simulink model "AE_BoltEV_LMDI"  (R2026a)
settings: Solver=ode23t  StartTime=0  StopTime=1800  FixedStep=Ts  MaxStep=0.01  EnableMultiTasking=on
InitFcn:
  | AE_BoltEV_LMDI_Params;
undefined symbols (not defined in the file): id_map, iq_map, Is_map, n_loss_bp, P, P_cu_map, P_iron_map, T_loss_bp, Tmax, V_oc
libraries: nesl_utility x14, fl_lib x12, autolibshared x2, sdl_lib x2, autolibmappedmotor x1, sl_discontinuities x1
(part 2 of 3)

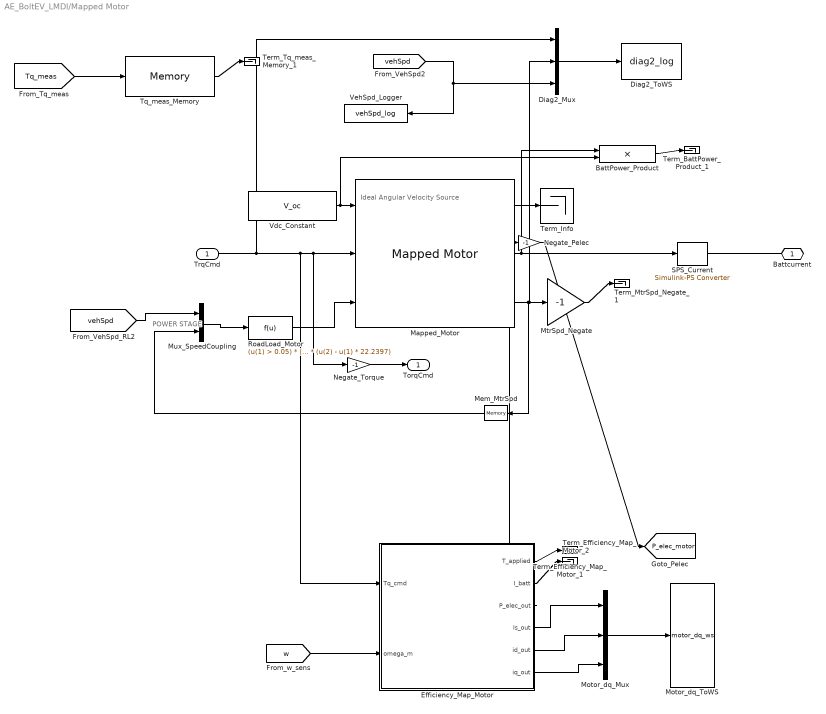
== system AE_BoltEV_LMDI/Mapped Motor ==
  note: Ideal Angular Velocity Source
  note: POWER STAGE
  TrqCmd : Inport
  BattPower_Product : Product
  Diag2_Mux : Mux  Inputs=3
  Diag2_ToWS : ToWorkspace  VariableName=diag2_log  SampleTime=0.1
  Efficiency_Map_Motor : Subsystem  Description=Efficiency-map motor. P_elec = sign(Tw)(|Tw| + P_loss). Bolt EV 150 kW IPM.
  Mapped_Motor : autolibmappedmotor/Mapped Motor  w_Tmax_bp_ext=[-921.533845053006 -837.758040957278 -785.398163397448 -733.038285837618 -680.678408277789 -628.318530717959 -575.958653158129 -523.598775598299 -460.766922526503 -366.519142918809 -0.10471975511966 0 0.10471975511966 366.519142918809 460.766922526503 523.598775598299 575.958653158129 628.318530717959 680.678408277789 733.038285837618 785.398163397448 837.758040957278 921.533845053006]  Tmax_w_V_ext=[162 162 162;179 179 179;191 191 191;204 204 204;220 220 220;238 238 238;260 260 260;286 286 286;325 325 325;360 360 360;360 360 360;360 360 360;360 360 360;360 360 360;325 325 325;286 286 286;260 260 260;238 238 238;220 220 220;204 204 204;191 191 191;179 179 179;162 162 162]  w_Tmin_bp_ext=[-921.533845053006 -837.758040957278 -785.398163397448 -733.038285837618 -680.678408277789 -628.318530717959 -575.958653158129 -523.598775598299 -460.766922526503 -366.519142918809 -0.10471975511966 0 0.10471975511966 366.519142918809 460.766922526503 523.598775598299 575.958653158129 628.318530717959 680.678408277789 733.038285837618 785.398163397448 837.758040957278 921.533845053006]  Tmin_w_V_ext=[-162 -162 -162;-179 -179 -179;-191 -191 -191;-204 -204 -204;-220 -220 -220;-238 -238 -238;-260 -260 -260;-286 -286 -286;-325 -325 -325;-360 -360 -360;-360 -360 -360;-360 -360 -360;-360 -360 -360;-360 -360 -360;-325 -325 -325;-286 -286 -286;-260 -260 -260;-238 -238 -238;-220 -220 -220;-204 -204 -204;-191 -191 -191;-179 -179 -179;-162 -162 -162]  port_config=Torque  param_by=Tabulated torque-speed envelope  w_t=[0 0.10471975511966 366.519142918809 460.766922526503 523.598775598299 575.958653158129 628.318530717959 680.678408277789 733.038285837618 785.398163397448 837.758040957278 921.533845053006]  T_t=[360 360 360 325 286 260 238 220 204 191 179 162]  torque_max=360  power_max=150  SpreadsheetTqLimitsFileName=MotorCalibrationImportData.xlsx  Tmax_w_V=[360 360 360;360 360 360;360 360 360;325 325 325;286 286 286;260 260 260;238 238 238;220 220 220;204 204 204;191 191 191;179 179 179;162 162 162]  w_Tmax_bp=[0 0.10471975511966 366.519142918809 460.766922526503 523.598775598299 575.958653158129 628.318530717959 680.678408277789 733.038285837618 785.398163397448 837.758040957278 921.533845053006]  V_Tmax_bp=[300 380 420]  Tmin_w_V=[-360 -360 -360;-360 -360 -360;-360 -360 -360;-325 -325 -325;-286 -286 -286;-260 -260 -260;-238 -238 -238;-220 -220 -220;-204 -204 -204;-191 -191 -191;-179 -179 -179;-162 -162 -162]  w_Tmin_bp=[0 0.10471975511966 366.519142918809 460.766922526503 523.598775598299 575.958653158129 628.318530717959 680.678408277789 733.038285837618 785.398163397448 837.758040957278 921.533845053006]  V_Tmin_bp=[300 380 420]  Tc=0.02  param_loss=Tabulated loss data  SpreadsheetLossFileName=MotorCalibrationImportData.xlsx  SpreadsheetEffFileName=MotorCalibrationImportData.xlsx  eff=100  w_eff=375  T_eff=0.08  Piron=0  Pbase=0  w_eff_bp=[10.472 31.4159 52.3599 73.3038 94.2478 115.192 136.136 157.08 178.024 198.968 219.911 240.855 261.799 282.743 303.687 324.631 345.575 366.519 387.463 408.407 429.351 450.295 471.239 492.183 513.127 534.071 555.015 575.959 596.903 617.847 638.791 659.734 680.678 701.622 722.566 743.51 764.454 785.398 806.342 827.286 848.23 869.174 890.118 911.062]  T_eff_bp=[5 15 25 35 45 55 65 75 85 95 105 115 125 135 145 155 165 175 185 195 205 215 225 235 245 255 265 275 285 295 305 315 325 335 345 355]  Temp_eff_bp=[233.15 293.15 373.15]  V_eff_bp=[500 700 900]  losses_table=[0.0510406 0.0625521 0.178396 0.24029 0.27318 0.319399 0.278867 0.4974 0.605444 0.760038 0.914632 0.914632 0.914632 0.914632 0.914632 0.914632 0.914632 0.914632 0.914632 0.914632 0.914632 0.914632 0.914632 0.914632 0.914632 0.914632 0.914632 0.914632 0.914632 0.914632 0.914632 0.914632 0.914632 0.914632 0.914632 0.914632;0.0638076 0.134097 0.288464 0.442831 0.442198 0.435705 0.564537 0.583406 0.63604 0.705391 0.960056 0.79415 1.15198 1.85898 1.15198 1.15198 1.15198 1.15198 1.15198 1.15198 1.15198 1.15198 1.15198 1.15198 1.15198 1.15198 1.15198 1.15198 1.15198 1.15198 1.15198 1.15198 1.15198 1.15198 1.15198 1.15198;0.180074 0.242567 0.34561 0.494816 0.644021 0.731051 0.678035 0.649813 0.985578 1.08383 1.11012 1.13567 1.46263 1.79781 2.13298 2.46815 2.80332 3.51032 1.46263 1.46263 1.46263 1.46263 1.46263 1.46263 1.46263 1.46263 1.46263 1.46263 1.46263 1.46263 1.46263 1.46263 1.46263 1.46263 1.46263 1.46263;0.169987 0.286066 0.402144 0.518223 0.667751 0.81728 0.966809 0.773099 0.990937 1.17316 1.38469 1.25266 1.46877 1.86485 2.26092 2.657 3.05307 3.44915 3.78432 4.11949 4.45466 5.16166 1.46877 1.46877 1.46877 1.46877 1.46877 1.46877 1.46877 1.46877 1.46877 1.46877 1.46877 1.46877 1.46877 1.46877;0.150576 0.228366 0.479817 0.499144 0.609253 0.950688 0.944754 0.902321 1.21988 1.38258 1.52287 1.54298 1.63876 2.01026 2.38176 2.75325 3.12475 3.49625 3.86775 4.24744 4.64351 5.03959 5.43566 5.77083 6.106 1.63876 1.63876 1.63876 1.63876 1.63876 1.63876 1.63876 1.63876 1.63876 1.63876 1.63876;0.252548 0.419793 0.455765 0.661303 0.866841 0.913095 1.05779 1.29872 1.389 1.31786 1.63888 1.91867 1.79245 2.16558 2.5387 2.91183 3.28496 3.65809 4.03121 4.40434 4.77747 5.1506 5.52372 5.89522 6.26672 6.63822 7.0261 7.42217 7.75735 1.79245 1.79245 1.79245 1.79245 9.40869 9.40869 9.40869;0.373019 0.390819 0.133584 0.05 0.830136 0.973701 1.23193 1.22934 1.13798 1.46279 1.78761 1.88598 1.7209 1.57806 2.50827 2.84976 3.19125 3.53273 3.87422 4.21571 4.55719 4.89868 5.24017 5.58165 5.92314 6.26462 6.37758 6.49053 6.82226 7.154 7.48573 7.62379 9.40869 9.40869 9.40869 9.40869;0.394844 0.373616 0.770605 0.800456 0.811841 0.936385 1.23068 1.31503 1.39273 2.22246 1.97453 1.9104 2.04383 2.35679 2.62119 2.88558 3.14997 3.41437 3.67876 3.94315 4.20755 4.47194 4.73633 5.00072 5.26512 5.52951 5.7939 6.0583 6.36111 6.66392 6.96673 7.52277 7.52277 7.52277 7.52277 7.52277;0.368168 0.355256 0.465313 0.7562 0.810534 1.0698 1.27488 1.38255 1.48307 1.82538 2.21139 2.43878 2.31392 2.57641 2.8389 3.10138 3.36387 3.62636 3.88885 4.15134 4.41383 4.67632 4.93881 5.2013 5.46378 5.72627 5.98876 6.25125 6.51374 6.77623 7.03872 7.30121 2.31392 7.52277 7.52277 7.52277;0.202464 0.449991 0.765628 0.745597 0.834475 1.10068 1.33495 1.47005 1.68039 1.74236 2.38963 2.74438 2.2255 2.46609 2.70668 2.94727 3.18786 3.42845 3.66904 3.90963 4.15022 4.39081 4.6314 4.87199 5.11258 5.35317 5.59376 5.83435 6.07494 6.31553 6.69758 7.07964 7.07964 7.07964 7.07964 7.07964;0.385182 0.539154 0.73648 0.73773 0.951019 1.23197 1.42671 1.74835 1.78431 1.8178 2.59901 2.34892 2.44302 2.59091 2.73879 2.98183 3.22488 3.46792 3.71096 3.954 4.19705 4.44009 4.68313 4.92617 5.16921 5.41226 5.6553 5.95693 6.25855 6.56018 6.86181 7.16343 7.16343 7.16343 7.16343 7.16343;0.571043 0.67941 0.78616 0.814092 1.04217 1.26551 1.32901 1.73004 1.77653 2.04145 2.30637 2.29889 2.33964 2.5267 2.71375 2.96113 3.20851 3.45589 3.70326 3.95064 4.19802 4.4454 4.69277 4.94015 5.18753 5.43491 5.68228 6.24622 6.81016 7.3741 7.57399 8.09419 7.57399 7.57399 7.57399 7.57399;0.911104 0.877468 0.95014 1.05464 1.27459 1.3082 1.45668 1.61397 1.82358 2.03319 2.24279 2.16306 2.56471 2.87964 3.19456 3.50948 3.8244 4.13932 4.45424 4.76917 5.08409 5.39901 5.71393 6.02885 6.34378 6.6587 6.89692 7.13514 7.37336 7.61158 7.8498 9.02495 9.02495 9.02495 9.02495 9.02495;0.888105 0.961962 1.0084 1.10491 1.2956 1.22143 1.59547 1.63831 1.82582 2.01332 2.20083 1.99424 2.3068 2.72718 3.05456 3.38194 3.70932 4.0367 4.36408 4.69146 5.01884 5.34622 5.6736 ...(+8702 chars)]  losses_table_3d=cat(3,1.05*[1.49 1.67 2.21 3.10; 0.42 0.69 1.14 2.03; 0.06 0.24 0.78 1.68; 0.42 0.69 1.14 2.03; 1.49 1.67 2.21 3.10],[1.49 1.67 2.21 3.10; 0.42 0.69 1.14 2.03; 0.06 0.24 0.78 1.68; 0.42 0.69 1.14 2.03; 1.49 1.67 2.21 3.10],1.03*[1.49 1.67 2.21 3.10; 0.42 0.69 1.14 2.03; 0.06 0.24 0.78 1.68; 0.42 0.69 1.14 2.03; 1.49 1.67 2.21 3.10])  losses_table_4d=cat(4,cat(3,[1.5645 0.441 0.063 0.441 1.5645;1.7535 0.7245 0.252 0.7245 1.7535;2.3205 1.197 0.819 1.197 2.3205;3.255 2.1315 1.764 2.1315 3.255],[1.5645 0.441 0.063 0.441 1.5645;1.7535 0.7245 0.252 0.7245 1.7535;2.3205 1.197 0.819 1.197 2.3205;3.255 2.1315 1.764 2.1315 3.255],[1.5645 0.441 0.063 0.441 1.5645;1.7535 0.7245 0.252 0.7245 1.7535;2.3205 1.197 0.819 1.197 2.3205;3.255 2.1315 1.764 2.1315 3.255]),cat(3,[1.49 0.42 0.06 0.42 1.49;1.67 0.69 0.24 0.69 1.67;2.21 1.14 0.78 1.14 2.21;3.1 2.03 1.68 2.03 3.1],[1.49 0.42 0.06 0.42 1.49;1.67 0.69 0.24 0.69 1.67;2.21 1.14 0.78 1.14 2.21;3.1 2.03 1.68 2.03 3.1],[1.49 0.42 0.06 0.42 1.49;1.67 0.69 0.24 0.69 1.67;2.21 1.14 0.78 1.14 2.21;3.1 2.03 1.68 2.03 3.1]),cat(3,[1.5347 0.4326 0.0618 0.4326 1.5347;1.7201 0.7107 0.2472 0.7107 1.7201;2.2763 1.1742 0.8034 1.1742 2.2763;3.193 2.0909 1.7304 2.0909 3.193],[1.5347 0.4326 0.0618 0.4326 1.5347;1.7201 0.7107 0.2472 0.7107 1.7201;2.2763 1.1742 0.8034 1.1742 2.2763;3.193 2.0909 1.7304 2.0909 3.193],[1.5347 0.4326 0.0618 0.4326 1.5347;1.7201 0.7107 0.2472 0.7107 1.7201;2.2763 1.1742 0.8034 1.1742 2.2763;3.193 2.0909 1.7304 2.0909 3.193]))  efficiency_table=[95 95 95 95; 95 95 95 95; 95 95 95 95; 95 95 95 95; 95 95 95 95]  efficiency_table_3d=cat(3,90*ones(5,4),95*ones(5,4),92*ones(5,4))  efficiency_table_4d=cat(4,cat(3,90*ones(5,4)',90*ones(5,4)',90*ones(5,4)'),cat(3,95*ones(5,4)',95*ones(5,4)',95*ones(5,4)'),cat(3,92*ones(5,4)',92*ones(5,4)',92*ones(5,4)'))  J=100  b=0.001  omega_o=0  T_t_extended=[162 179 191 204 220 238 260 286 325 360 360 360 360 360 325 286 260 238 220 204 191 179 162]  w_t_extended=[-921.533845053006 -837.758040957278 -785.398163397448 -733.038285837618 -680.678408277789 -628.318530717959 -575.958653158129 -523.598775598299 -460.766922526503 -366.519142918809 -0.10471975511966 0 0.10471975511966 366.519142918809 460.766922526503 523.598775598299 575.958653158129 628.318530717959 680.678408277789 733.038285837618 785.398163397448 837.758040957278 921.533845053006]  KLossIron=0  KLossCopper=0  x_w_eff_vec=[-911.062 -890.118 -869.174 -848.23 -827.286 -806.342 -785.398 -764.454 -743.51 -722.566 -701.622 -680.678 -659.734 -638.791 -617.847 -596.903 -575.959 -555.015 -534.071 -513.127 -492.183 -471.239 -450.295 -429.351 -408.407 -387.463 -366.519 -345.575 -324.631 -303.687 -282.743 -261.799 -240.855 -219.911 -198.968 -178.024 -157.08 -136.136 -115.192 -94.2478 -73.3038 -52.3599 -31.4159 10.472 31.4159 52.3599 73.3038 94.2478 115.192 136.136 157.08 178.024 198.968 219.911 240.855 261.799 282.743 303.687 324.631 345.575 366.519 387.463 408.407 429.351 450.295 471.239 492.183 513.127 534.071 555.015 575.959 596.903 617.847 638.791 659.734 680.678 701.622 722.566 743.51 764.454 785.398 806.342 827.286 848.23 869.174 890.118 911.062]  x_T_eff_vec=[-355 -345 -335 -325 -315 -305 -295 -285 -275 -265 -255 -245 -235 -225 -215 -205 -195 -185 -175 -165 -155 -145 -135 -125 -115 -105 -95 -85 -75 -65 -55 -45 -35 -25 -15 5 15 25 35 45 55 65 75 85 95 105 115 125 135 145 155 165 175 185 195 205 215 225 235 245 255 265 275 285 295 305 315 325 335 345 355]  x_tmp_eff_vec=[233.15 293.15 373.15]  x_V_eff_vec=[500 700 900]  x_losses_mat=[14.7373 14.7373 14.7373 14.7373 14.7373 14.7373 14.7373 14.7373 14.7373 14.7373 14.7373 14.7373 14.7373 14.7373 14.7373 14.7373 14.7373 14.7373 14.7373 14.7373 15.4019 15.4019 15.4019 15.4019 5.16995 5.16995 5.16995 5.16995 5.16995 3.05067 3.05067 55.8218 55.8218 55.8218 0.673171 0.673171 0.673171 55.8218 55.8218 55.8218 3.05067 3.05067 5.16995 5.16995 5.16995 5.16995 5.16995 15.4019 15.4019 15.4019 15.4019 14.7373 14.7373 14.7373 14.7373 14.7373 14.7373 14.7373 14.7373 14.7373 14.7373 14.7373 14.7373 14.7373 14.7373 14.7373 14.7373 14.7373 14.7373 14.7373 14.7373;14.7373 14.7373 14.7373 14.7373 14.7373 14.7373 14.7373 14.7373 14.7373 14.7373 14.7373 14.7373 14.7373 14.7373 14.7373 14.7373 14.7373 14.7373 14.7373 14.7373 15.4019 15.4019 15.4019 15.4019 5.16995 5.16995 5.16995 5.16995 5.16995 3.05067 3.05067 55.8218 55.8218 55.8218 0.673171 0.673171 0.673171 55.8218 55.8218 55.8218 3.05067 3.05067 5.16995 5.16995 5.16995 5.16995 5.16995 15.4019 15.4019 15.4019 15.4019 14.7373 14.7373 14.7373 14.7373 14.7373 14.7373 14.7373 14.7373 14.7373 14.7373 14.7373 14.7373 14.7373 14.7373 14.7373 14.7373 14.7373 14.7373 14.7373 14.7373;14.7373 14.7373 14.7373 14.7373 14.7373 14.7373 14.7373 14.7373 14.7373 14.7373 14.7373 14.7373 14.7373 14.7373 14.7373 14.7373 14.7373 14.7373 14.7373 14.7373 15.4019 15.4019 15.4019 15.4019 5.16995 5.16995 5.16995 5.16995 5.16995 3.05067 3.05067 55.8218 55.8218 55.8218 0.673171 0.673171 0.673171 55.8218 55.8218 55.8218 3.05067 3.05067 5.16995 5.16995 5.16995 5.16995 5.16995 15.4019 15.4019 15.4019 15.4019 14.7373 14.7373 14.7373 14.7373 14.7373 14.7373 14.7373 14.7373 14.7373 14.7373 14.7373 14.7373 14.7373 14.7373 14.7373 14.7373 14.7373 14.7373 14.7373 14.7373;14.7373 14.7373 14.7373 14.7373 14.7373 14.7373 14.7373 14.7373 14.7373 14.7373 14.7373 14.7373 14.7373 14.7373 14.7373 14.7373 14.7373 14.7373 14.7373 14.7373 15.4019 15.4019 15.4019 15.4019 5.16995 5.16995 5.16995 5.16995 5.16995 3.05067 3.05067 55.8218 55.8218 55.8218 0.673171 0.673171 0.673171 55.8218 55.8218 55.8218 3.05067 3.05067 5.16995 5.16995 5.16995 5.16995 5.16995 15.4019 15.4019 15.4019 15.4019 14.7373 14.7373 14.7373 14.7373 14.7373 14.7373 14.7373 14.7373 14.7373 14.7373 14.7373 14.7373 14.7373 14.7373 14.7373 14.7373 14.7373 14.7373 14.7373 14.7373;14.7373 14.7373 14.7373 14.7373 14.7373 14.7373 14.7373 14.7373 14.7373 14.7373 14.7373 14.7373 14.7373 14.7373 14.7373 14.7373 14.7373 14.7373 14.7373 14.7373 15.4019 13.9402 12.4785 11.0168 9.55505 8.09335 6.63165 5.16995 4.46352 3.7571 3.05067 55.8218 46.6304 37.4389 28.2475 19.0561 28.2475 37.4389 46.6304 55.8218 3.05067 3.7571 4.46352 5.16995 6.63165 8.09335 9.55505 11.0168 12.4785 13.9402 15.4019 14.7373 14.7373 14.7373 14.7373 14.7373 14.7373 14.7373 14.7373 14.7373 14.7373 14.7373 14.7373 14.7373 14.7373 14.7373 14.7373 14.7373 14.7373 14.7373 14.7373;15.0311 15.0311 15.0311 15.0311 15.0311 15.0311 15.0311 15.0311 15.0311 15.0311 15.0311 15.0311 15.0311 15.0311 15.0311 15.0311 15.0311 15.0311 15.0311 15.0311 15.234 12.7976 10.3613 9.34045 8.31962 7.29879 6.27796 5.25713 4.12058 3.24271 2.61916 2.846 1.91391 10.7458 19.5776 28.4095 19.5776 10.7458 1.91391 2.846 2.61916 3.24271 4.12058 5.25713 6.27796 7.29879 8.31962 9.34045 10.3613 12.7976 15.234 15.0311 15.0311 15.0311 15.0311 15.0311 15.0311 15.0311 15.0311 15.0311 15.0311 15.0311 15.0311 15.0311 15.0311 15.0311 15.0311 15.0311 15.0311 15.0311 15.0311;15.1554 15.1554 15.1554 15.1554 15.1554 15.1554 15.1554 15.1554 15.1554 15.1554 15.1554 15.1554 15.1554 15.1554 15.1554 15.1554 15.1554 15.1554 15.1554 15.2236 13.795 12.3665 10.938 9.50943 8.08089 6.65235 5.22381 4.60929 3.99478 3.12888 2.34087 2.09005 1.83923 1.60864 1.37804 1.14745 1.37804 1.60864 1.83923 2.09005 2.34087 3.12888 3.99478 4.60929 5.22381 6.65235 8.08089 9.50943 10.938 12.3665 13.795 15.2236 15.1554 15.1554 15.1554 15.1554 15.1554 15.1554 15.1554 15.1554 15.1554 15.1554 15.1554 15.1554 15.1554 15.1554 15.1554 15.1554 15.1554 15.1554 15.1554;15.2061 15.2061 ...(+45376 chars)]  x_losses_mat_3d=cat(3,[3.255 2.3205 1.7535 1.5645 1.7535 2.3205 3.255;2.1315 1.197 0.7245 0.441 0.7245 1.197 2.1315;1.764 0.819 0.252 0.063 0.252 0.819 1.764;2.1315 1.197 0.7245 0.441 0.7245 1.197 2.1315;3.255 2.3205 1.7535 1.5645 1.7535 2.3205 3.255],[3.1 2.21 1.67 1.49 1.67 2.21 3.1;2.03 1.14 0.69 0.42 0.69 1.14 2.03;1.68 0.78 0.24 0.06 0.24 0.78 1.68;2.03 1.14 0.69 0.42 0.69 1.14 2.03;3.1 2.21 1.67 1.49 1.67 2.21 3.1],[3.193 2.2763 1.7201 1.5347 1.7201 2.2763 3.193;2.0909 1.1742 0.7107 0.4326 0.7107 1.1742 2.0909;1.7304 0.8034 0.2472 0.0618 0.2472 0.8034 1.7304;2.0909 1.1742 0.7107 0.4326 0.7107 1.1742 2.0909;3.193 2.2763 1.7201 1.5347 1.7201 2.2763 3.193])  x_losses_mat_4d="reshape([80;53.33;26.67;0;24;48;72;40;26.67;13.33;0;12;24;36;0;0;0;0;0;0;0;36;24;12;0;13.33;26.67;40;72;48;24;0;26.67;53.33;80;80;53.33;26.67;0;24;48;72;40;26.67;13.33;0;12;24;36;0;0;0;0;0;0;0;36;24;12;0;13.33;26.67;40;72;48;24;0;26.67;53.33;80;80;53.33;26.67;0;24;48;72;40;26.67;13.33;0;12;24;36;0;0;0;0;0;0;0;36;24;12;0;13.33;26.67;40;72;48;24;0;26.67;53.33;80;37.89;25.26;12.63;0;12;24;36;18.95;12.63;6.32;0;6;12;18;0;0;0;0;0;0;0;18;12;6;0;6.32;12.63;18.95;36;24;12;0;12.63;25.26;37.89;37.89;25.26;12.63;0;12;24;36;18.95;12.63;6.32;0;6;12;18;0;0;0;0;0;0;0;18;12;6;0;6.32;12.63;18.95;36;24;12;0;12.63;25.26;37.89;37.89;25.26;12.63;0;12;24;36;18.95;12.63;6.32;0;6;12;18;0;0;0;0;0;0;0;18;12;6;0;6.32;12.63;18.95;36;24;12;0;12.63;25.26;37.89;62.61;41.74;20.87;0;19.2;38.4;57.6;31.3;20.87;10.43;0;9.6;19.2;28.8;0;0;0;0;0;0;0;28.8;19.2;9.6;0;10.43;20.87;31.3;57.6;38.4;19.2;0;20.87;41.74;62.61;62.61;41.74;20.87;0;19.2;38.4;57.6;31.3;20.87;10.43;0;9.6;19.2;28.8;0;0;0;0;0;0;0;28.8;19.2;9.6;0;10.43;20.87;31.3;57.6;38.4;19.2;0;20.87;41.74;62.61;62.61;41.74;20.87;0;19.2;38.4;57.6;31.3;20.87;10.43;0;9.6;19.2;28.8;0;0;0;0;0;0;0;28.8;19.2;9.6;0;10.43;20.87;31.3;57.6;38.4;19.2;0;20.87;41.74;62.61], [7  5  3  3])"  CalLossMapData={}  CalLossWithTempMapData={}  aMode=1  RefBlkName='autolibmappedmotor/Mapped Motor'
      settings: LibrarySourceBlock=autolibemachines/Mapped Motor
  Mem_MtrSpd : Memory
  Motor_dq_Mux : Mux  Inputs=3
  Motor_dq_ToWS : ToWorkspace  VariableName=motor_dq_ws  SaveFormat=Structure With Time  SampleTime=-1
  MtrSpd_Negate : Gain  Gain=-1
  Mux_SpeedCoupling : Mux  Inputs=2
  Negate_Pelec : Gain  Gain=-1
  Negate_Torque : Gain  Gain=-1
  RoadLoad_Motor : Fcn  Expr=(u(1) > 0.05) * (126.3 + 2.008*u(1) + 0.4336*u(1)*u(1)) * 0.3170 / 7.05 + -1000.0 * (u(2) - u(1) * 22.2397)
  SPS_Current : nesl_utility/Simulink-PS Converter  PhysicalDomain=network_engine_domain  SubClassName=ps_input  LeftPortType=input  RightPortType=output  PseudoPeriodic=off  Frequencies=[]  NoiseDistribution=none  NoiseParameters=[]  Unit=A  AffineConversion=off  FilteringAndDerivatives=provide  SimscapeFilterOrder=1  InputFilterTimeConstant=0.001  UdotUserProvided=0
  Term_BattPower_Product_1 : Terminator
  Term_Efficiency_Map_Motor_1 : Terminator
  Term_Efficiency_Map_Motor_2 : Terminator
  Term_Info : Terminator
  Term_MtrSpd_Negate_1 : Terminator
  Term_Tq_meas_Memory_1 : Terminator
  Tq_meas_Memory : Memory
  Vdc_Constant : Constant  Value=V_oc  OutDataTypeStr=double
  VehSpd_Logger : ToWorkspace  VariableName=vehSpd_log  SampleTime=0.1
  Battcurrent : PMIOPort  Side=Right
  TorqCmd : Outport
  tag scope: P_elec_motor=global
  wires:
  RoadLoad_Motor/1 -> Mapped_Motor/3
  Efficiency_Map_Motor/2(I_batt) -> Term_Efficiency_Map_Motor_2/1
  BattPower_Product/1 -> Term_BattPower_Product_1/1
  [w] -> Efficiency_Map_Motor/2(omega_m)
  Efficiency_Map_Motor/5(id_out) -> Motor_dq_Mux/2
  Efficiency_Map_Motor/6(iq_out) -> Motor_dq_Mux/3
  Efficiency_Map_Motor/1(T_applied) -> Term_Efficiency_Map_Motor_1/1
  TrqCmd/1 -> Negate_Torque/1, Mapped_Motor/2, Efficiency_Map_Motor/1(Tq_cmd), Diag2_Mux/1
  Mem_MtrSpd/1 -> Mux_SpeedCoupling/2
  Mux_SpeedCoupling/1 -> RoadLoad_Motor/1
  Mapped_Motor/1 -> Term_Info/1
  MtrSpd_Negate/1 -> Term_MtrSpd_Negate_1/1
  Mapped_Motor/2 -> BattPower_Product/1, SPS_Current/1
  [Tq_meas] -> Tq_meas_Memory/1
  Vdc_Constant/1 -> Mapped_Motor/1, BattPower_Product/2
  Diag2_Mux/1 -> Diag2_ToWS/1
  Efficiency_Map_Motor/4(Is_out) -> Motor_dq_Mux/1
  Negate_Torque/1 -> TorqCmd/1
  [vehSpd] -> Diag2_Mux/3, VehSpd_Logger/1
  [vehSpd] -> Mux_SpeedCoupling/1
  Motor_dq_Mux/1 -> Motor_dq_ToWS/1
  Tq_meas_Memory/1 -> Term_Tq_meas_Memory_1/1
  Mapped_Motor/3 -> MtrSpd_Negate/1, Diag2_Mux/2, Mem_MtrSpd/1
  Efficiency_Map_Motor/3(P_elec_out) -> Negate_Pelec/1
  Negate_Pelec/1 -> [P_elec_motor]
  connections:
  SPS_Current/RConn1 -- Battcurrent/RConn1
